simulink model "FrictionTest"  (Simulink 7.9)
settings: Solver=ode3  StartTime=0.0  StopTime=8  RelTol=1e-3
undefined symbols (not defined in the file or in its folder): DiscIntNeverNeededParam
libraries: simulink x5
settings Model: Creator=Administrator  LastModifiedBy=Administrator

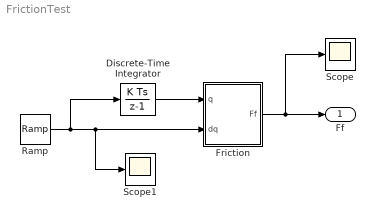
== system FrictionTest ==
  Discrete-Time Integrator : DiscreteIntegrator  SampleTime=0.00025  ICPrevOutput=DiscIntNeverNeededParam  ICPrevScaledInput=DiscIntNeverNeededParam
  Friction : Subsystem  mask{Ts=0.00025, FpSelect=1}
      mask prompts: Ts "Sampling Time"
  Ramp : simulink/Sources/Ramp  slope=50  start=0  X0=-200
  Scope : Scope
      settings: YMin=320  YMax=500  SaveName=Ff
  Scope1 : Scope
      settings: SaveName=dq
  Ff : Outport
  wires:
  Friction/1(Ff) -> Scope/1, Ff/1
  Ramp/1 -> Discrete-Time Integrator/1, Scope1/1, Friction/2(dq)
  Discrete-Time Integrator/1 -> Friction/1(q)

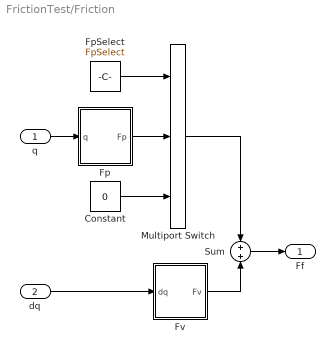
== system FrictionTest/Friction ==
  q : Inport
  dq : Inport  Port=2
  Constant : Constant  Value=0  SampleTime=Ts
  Fp : Subsystem  mask{Ts=Ts, B1=-0.0052, B2=0.0018, B3=0.0024, B4=-0.0092}
      mask prompts: Ts "Sampling Time"
  FpSelect : Constant  Value=FpSelect  SampleTime=Ts
  Fv : Subsystem  mask{Ts=Ts, fc=0.0194, fs=0.0293, lamda=2, theta=0.000013, dqs=55.219}
      mask prompts: Ts "Sampling Time"
  Multiport Switch : MultiPortSwitch  Inputs=2  zeroidx=off  SampleTime=Ts
  Sum : Sum  Inputs=+|+  SampleTime=Ts
  Ff : Outport
  wires:
  q/1 -> Fp/1(q)
  dq/1 -> Fv/1(dq)
  Fv/1(Fv) -> Sum/2
  Sum/1 -> Ff/1
  Multiport Switch/1 -> Sum/1
  Fp/1(Fp) -> Multiport Switch/2
  Constant/1 -> Multiport Switch/3
  FpSelect/1 -> Multiport Switch/1

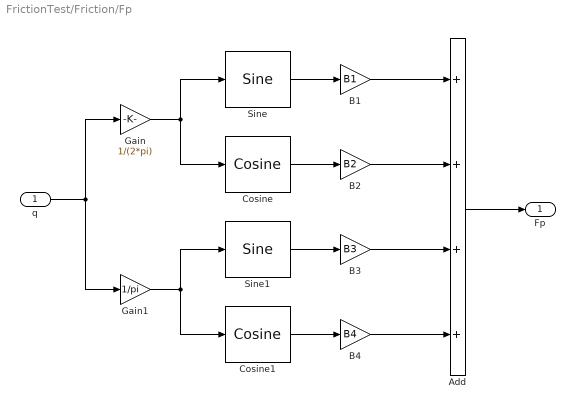
== system FrictionTest/Friction/Fp ==
  q : Inport
  Add : Sum  Inputs=++++  SampleTime=Ts
  B1 : Gain  Gain=B1  SampleTime=Ts
  B2 : Gain  Gain=B2  SampleTime=Ts
  B3 : Gain  Gain=B3  SampleTime=Ts
  B4 : Gain  Gain=B4  SampleTime=Ts
  Cosine : simulink/Lookup Tables/Cosine  Formula=cos(2*pi*u)  NumDataPoints=(2^5)+1  OutputWordLength=16
  Cosine1 : simulink/Lookup Tables/Cosine  Formula=cos(2*pi*u)  NumDataPoints=(2^5)+1  OutputWordLength=16
  Gain : Gain  Gain=1/(2*pi)  SampleTime=Ts
  Gain1 : Gain  Gain=1/pi  SampleTime=Ts
  Sine : simulink/Lookup Tables/Sine  Formula=sin(2*pi*u)  NumDataPoints=(2^5)+1  OutputWordLength=16
  Sine1 : simulink/Lookup Tables/Sine  Formula=sin(2*pi*u)  NumDataPoints=(2^5)+1  OutputWordLength=16
  Fp : Outport
  wires:
  Gain/1 -> Sine/1, Cosine/1
  Gain1/1 -> Sine1/1, Cosine1/1
  q/1 -> Gain/1, Gain1/1
  Cosine1/1 -> B4/1
  Sine1/1 -> B3/1
  Cosine/1 -> B2/1
  Sine/1 -> B1/1
  B2/1 -> Add/2
  B3/1 -> Add/3
  B4/1 -> Add/4
  B1/1 -> Add/1
  Add/1 -> Fp/1

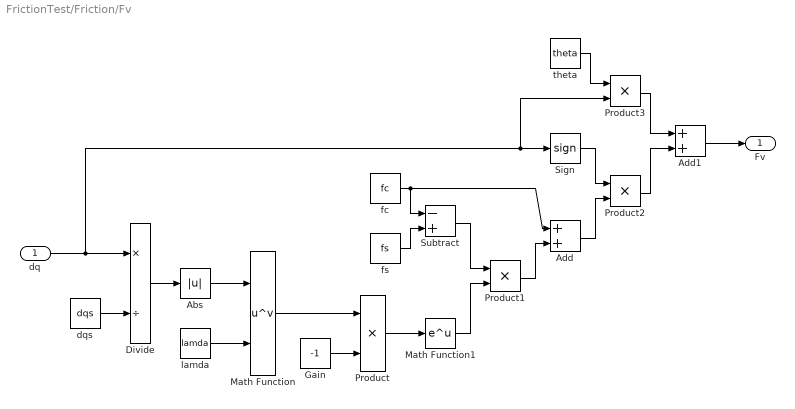
== system FrictionTest/Friction/Fv ==
  dq : Inport
  Abs : Abs  SampleTime=Ts
  Add : Sum  SampleTime=Ts
  Add1 : Sum  SampleTime=Ts
  Divide : Product  Inputs=*/  SampleTime=Ts
  Gain : Constant  Value=-1  SampleTime=Ts
  Math Function : Math  Operator=pow  SampleTime=Ts  SaturateOnIntegerOverflow=on
  Math Function1 : Math  SampleTime=Ts  SaturateOnIntegerOverflow=on
  Product{,1..3} (4 alike) : Product  SampleTime=Ts  RndMeth=Zero
  Sign : Signum  SampleTime=Ts
  Subtract : Sum  Inputs=-+  SampleTime=Ts
  dqs : Constant  Value=dqs  SampleTime=Ts
  fc : Constant  Value=fc  SampleTime=Ts
  fs : Constant  Value=fs  SampleTime=Ts
  lamda : Constant  Value=lamda  SampleTime=Ts
  theta : Constant  Value=theta  SampleTime=Ts
  Fv : Outport
  wires:
  dq/1 -> Divide/1, Sign/1, Product3/2
  dqs/1 -> Divide/2
  Divide/1 -> Abs/1
  Abs/1 -> Math Function/1
  lamda/1 -> Math Function/2
  Math Function/1 -> Product/1
  Gain/1 -> Product/2
  Product/1 -> Math Function1/1
  fc/1 -> Subtract/1, Add/1
  fs/1 -> Subtract/2
  Subtract/1 -> Product1/1
  Math Function1/1 -> Product1/2
  Product1/1 -> Add/2
  Sign/1 -> Product2/1
  Add/1 -> Product2/2
  Product3/1 -> Add1/1
  Product2/1 -> Add1/2
  theta/1 -> Product3/1
  Add1/1 -> Fv/1
